simulink model "Program_robot_control"  (R2020a)
settings: Solver=FixedStepAuto  StartTime=0.0  StopTime=10.0  RelTol=1e-3  EnableMultiTasking=on
libraries: legoev3lib x9, dspstat3 x1
settings Model: ExtModeTrigDuration=2  Creator=irene  LastModifiedBy=irene
settings SolverCC: PositivePriorityOrder=on
settings OptimizationCC: EnhancedBackFolding=on  PassReuseOutputArgsAs=Individual arguments  ZeroExternalMemoryAtStartup=off  ZeroInternalMemoryAtStartup=off  MaxStackSize=64  OptimizeBlockOrder=speed  DifferentSizesBufferReuse=on  OptimizationCustomize=off  EfficientTunableParamExpr=on
settings DebuggingCC: ParameterTunabilityLossMsg=error
settings HardwareCC: ProdBitPerPointer=32  ProdBitPerSizeT=32  ProdBitPerPtrDiffT=32  ProdLargestAtomicInteger=Long  ProdWordSize=32  ProdHWDeviceType=ARM Compatible->ARM 9  UseEmbeddedCoderFeatures=off  UseSimulinkCoderFeatures=off
settings SFSimCC: MATLABDynamicMemAlloc=off
settings RTWCC: SystemTargetFile=ert.tlc  HardwareBoard=LEGO MINDSTORMS EV3  TemplateMakefile=ert_default_tmf  Toolchain=Sourcery G++ Lite v2009q3
settings CodeAppCC: ForceParamTrailComments=on  IgnoreCustomStorageClasses=off  OperatorAnnotations=on  SimulinkDataObjDesc=on  SFDataObjDesc=on  InsertBlockDesc=on
settings ERTTargetCC: SupportContinuousTime=on  SupportNonInlinedSFcns=on  SupportVariableSizeSignals=on

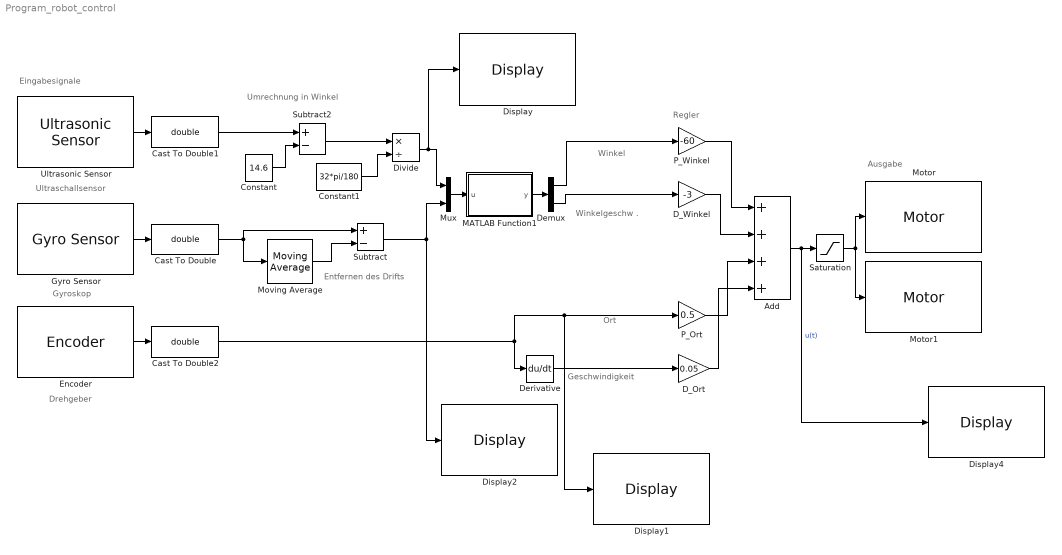
== system Program_robot_control ==
  note: Drehgeber
  note: Gyroskop
  note: Ultraschallsensor
  note: Winkel
  note: Winkelgeschw .
  note: Geschwindigkeit
  note: Ort
  note: Ausgabe
  note: Regler
  note: Entfernen des Drifts
  note: Umrechnung in Winkel
  note: Eingabesignale
  Add : Sum  Inputs=++++
  Cast To Double : DataTypeConversion  OutDataTypeStr=double
  Cast To Double1 : DataTypeConversion  OutDataTypeStr=double
  Cast To Double2 : DataTypeConversion  OutDataTypeStr=double
  Constant : Constant  Value=14.6
  Constant1 : Constant  Value=32*pi/180
  D_Ort : Gain  Gain=0.05
  D_Winkel : Gain  Gain=-3
  Demux : Demux  Outputs=2
  Derivative : Derivative
  Display : legoev3lib/Display  slcdStr=angle  slcdLine=2  slcdFormat=Decimal
      settings: SourceProductBaseCode=LEGOEV3
  Display1 : legoev3lib/Display  slcdStr=Ort  slcdLine=4  slcdFormat=Decimal
      settings: SourceProductBaseCode=LEGOEV3
  Display2 : legoev3lib/Display  slcdStr=Gyro o.D  slcdLine=3  slcdFormat=Decimal
      settings: SourceProductBaseCode=LEGOEV3
  Display4 : legoev3lib/Display  slcdStr=motor  slcdLine=5  slcdFormat=Decimal
      settings: SourceProductBaseCode=LEGOEV3
  Divide : Product  Inputs=*/
  Encoder : legoev3lib/Encoder  portNumber=C  opMode=No reset  sampleTime=0.01
      settings: SourceProductBaseCode=LEGOEV3
  Gyro Sensor : legoev3lib/Gyro Sensor  portNumber=4  sampleTime=0.01
      settings: SourceProductBaseCode=LEGOEV3
  MATLAB Function1 : MATLAB Function  TreatAsAtomicUnit=on
  Motor : legoev3lib/Motor  sportNumber=C  sstopAction=Brake
  Motor1 : legoev3lib/Motor  sportNumber=B  sstopAction=Brake
  Moving Average : dspstat3/Moving Average  Method=Exponential weighting  ForgettingFactorPort=off  SpecifyWindowLength=on  WindowLength=4  ForgettingFactor=0.9999  SimulateUsing=Code generation
  Mux : Mux  Inputs=2
  P_Ort : Gain  Gain=0.5
  P_Winkel : Gain  Gain=-60
  Saturation : Saturate  UpperLimit=100  LowerLimit=-100
  Subtract : Sum  Inputs=+-
  Subtract2 : Sum  Inputs=+-
  Ultrasonic Sensor : legoev3lib/Ultrasonic Sensor  PortNumber=2  sampleTime=0.01
      settings: SourceProductBaseCode=LEGOEV3
  wires:
  Cast To Double2/1 -> P_Ort/1, Display1/1, Derivative/1
  Subtract/1 -> Display2/1, Mux/2
  Subtract2/1 -> Divide/1
  Moving Average/1 -> Subtract/2
  Add/1 -> Display4/1, Saturation/1  "u(t)"
  Mux/1 -> MATLAB Function1/1(u)
  Gyro Sensor/1 -> Cast To Double/1
  Constant/1 -> Subtract2/2
  Encoder/1 -> Cast To Double2/1
  Cast To Double/1 -> Subtract/1, Moving Average/1
  Cast To Double1/1 -> Subtract2/1
  Ultrasonic Sensor/1 -> Cast To Double1/1
  Constant1/1 -> Divide/2
  Divide/1 -> Display/1, Mux/1
  MATLAB Function1/1(y) -> Demux/1
  Derivative/1 -> D_Ort/1
  Demux/2 -> D_Winkel/1
  Demux/1 -> P_Winkel/1
  P_Winkel/1 -> Add/1
  D_Winkel/1 -> Add/2
  P_Ort/1 -> Add/3
  D_Ort/1 -> Add/4
  Saturation/1 -> Motor1/1, Motor/1

== matlab function Program_robot_control/MATLAB Function1 ==
  data: u input; y output
function y = KalmanFilter(u)

persistent P00 P01 P10 P11 state0 state1
if isempty(P00) 
    P00 = 1000;
    P01 = 0;
    P10 = 0; 
    P11 = 1000;
    state0 = 0;
    state1 = 0;
end

meas0 = u(1);
meas1 = u(2);

dt = 0.01;
sig = 30;
an = 25;
apn = 25;

P00 = P00 + dt*(P01 + P10 + P11*dt + dt^3*sig^2/4);
P01 = P01 + dt*(P11 + dt^2*sig^2/2);
P10 = P10 + dt*(P11 + dt^2*sig^2/2);
P11 = P11 + dt^2*sig^2;
Sdet = P00*P11 + P00*apn^2 - P01*P10 + P11*an^2 + an^2*apn^2;
Sinv00 = (P11 + apn^2)/Sdet;
Sinv01 = -P01/Sdet;
Sinv10 = -P10/Sdet;
Sinv11 = (P00 + an^2)/Sdet;
K00 = P00*Sinv00 + P01*Sinv10;
K01 = P00*Sinv01 + P01*Sinv11;
K10 = P10*Sinv00 + P11*Sinv10;
K11 = P10*Sinv01 + P11*Sinv11;
w0 = meas0 - state0;
w1 = meas1 - state1;
state0 = K00*w0 + K01*w1 + dt*state1 + state0;
state1 = K10*w0 + K11*w1 + state1;
P00 = -K00*P00 - K01*P10 + P00;
P01 = -K00*P01 - K01*P11 + P01;
P10 = -K10*P00 - K11*P10 + P10;
P11 = -K10*P01 - K11*P11 + P11;

% Defines Output 
y = zeros(2,1);
y(1) = state0;
y(2) = state1;
